simulink model "ModelSpeedSolver"  (R2019b)
settings: Solver=VariableStepAuto  StartTime=0.0  StopTime=1  RelTol=1e-3
values from neighbouring files (symbols this model uses):
  envFactor = struct    [inputSolver.m]    (also in plotResult.m)
  T0 = 26    [inputSolver.m]
  V0 = 0/3.6    (= 0)    [inputSolver.m]
undefined symbols (not defined in the file or in its folder): modelPara, solverinput, Tfmax, Tfmin, Vfmax, Vfmin
settings Model: Creator=j9002  LastModifiedBy=j9002
settings DataIOCC: ReturnWorkspaceOutputs=off
settings DebuggingCC: ArithmeticOperatorsInVariantConditions=warning
settings SFSimCC: SimUseLocalCustomCode=off  CustomCodeUndefinedFunction=UseInterfaceOnly
settings RTWCC: RTWUseLocalCustomCode=off

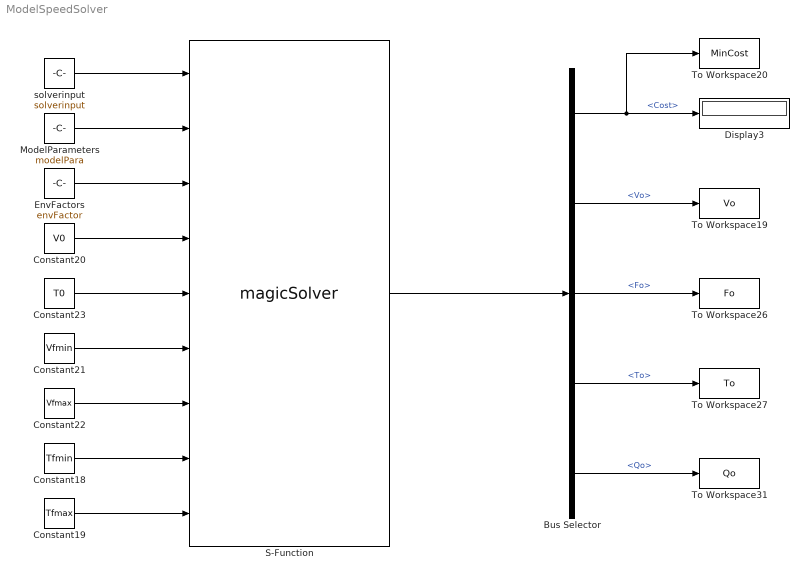
== system ModelSpeedSolver ==
  Bus Selector : BusSelector  OutputSignals=Cost,Vo,Fo,To,Qo
  Constant18 : Constant  Value=Tfmin
  Constant19 : Constant  Value=Tfmax
  Constant20 : Constant  Value=V0
  Constant21 : Constant  Value=Vfmin
  Constant22 : Constant  Value=Vfmax
  Constant23 : Constant  Value=T0
  Display3 : Display
  EnvFactors : Constant  Value=envFactor  OutDataTypeStr=Bus: EnvFactor
  ModelParameters : Constant  Value=modelPara  OutDataTypeStr=Bus: DynParameter
  S-Function : S-Function  FunctionName=magicSolver  SFunctionDeploymentMode=off  EnableBusSupport=off
  To Workspace19 : ToWorkspace  VariableName=Vo  SampleTime=-1
  To Workspace20 : ToWorkspace  VariableName=MinCost  SampleTime=-1
  To Workspace26 : ToWorkspace  VariableName=Fo  SampleTime=-1
  To Workspace27 : ToWorkspace  VariableName=To  SampleTime=-1
  To Workspace31 : ToWorkspace  VariableName=Qo  SampleTime=-1
  solverinput : Constant  Value=solverinput  OutDataTypeStr=Bus: SolverInput
  wires:
  S-Function/1 -> Bus Selector/1
  Bus Selector/4 -> To Workspace27/1  "<To>"
  Bus Selector/3 -> To Workspace26/1  "<Fo>"
  Bus Selector/1 -> Display3/1, To Workspace20/1  "<Cost>"
  Bus Selector/5 -> To Workspace31/1  "<Qo>"
  Bus Selector/2 -> To Workspace19/1  "<Vo>"
  ModelParameters/1 -> S-Function/2
  Constant19/1 -> S-Function/9
  EnvFactors/1 -> S-Function/3
  Constant20/1 -> S-Function/4
  Constant23/1 -> S-Function/5
  Constant22/1 -> S-Function/7
  Constant18/1 -> S-Function/8
  solverinput/1 -> S-Function/1
  Constant21/1 -> S-Function/6
